simulink model "Vehicle_kinematics_model"  (R2017b)
settings: Solver=FixedStepAuto  StartTime=0.0  StopTime=10.0  FixedStep=0.01  RelTol=1e-3
settings Model: Creator=18428  LastModifiedBy=18428

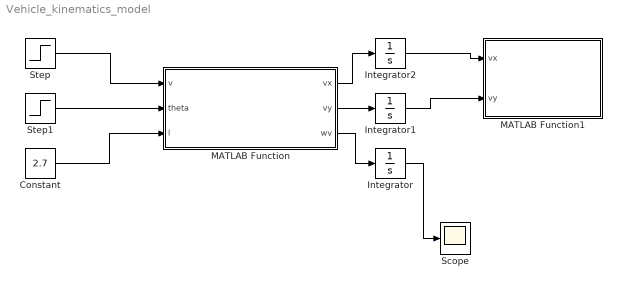
== system Vehicle_kinematics_model ==
  Constant : Constant  Value=2.7
  Integrator : Integrator
  Integrator1 : Integrator
  Integrator2 : Integrator
  MATLAB Function : MATLAB Function  TreatAsAtomicUnit=on
  MATLAB Function1 : MATLAB Function  TreatAsAtomicUnit=on
  Scope : Scope
  Step : Step  Time=0  After=5  SampleTime=0
  Step1 : Step  After=45  SampleTime=0
  wires:
  Step1/1 -> MATLAB Function/2(theta)
  Step/1 -> MATLAB Function/1(v)
  Constant/1 -> MATLAB Function/3(l)
  MATLAB Function/3(wv) -> Integrator/1
  Integrator/1 -> Scope/1
  MATLAB Function/2(vy) -> Integrator1/1
  MATLAB Function/1(vx) -> Integrator2/1
  Integrator2/1 -> MATLAB Function1/1(vx)
  Integrator1/1 -> MATLAB Function1/2(vy)

== matlab function Vehicle_kinematics_model/MATLAB Function1 ==
  data: vx input; vy input
function display_v(vx,vy)
    plot(vx,vy,'*');
    hold on
end

== matlab function Vehicle_kinematics_model/MATLAB Function ==
  data: v input; vx output; theta input; l input; vy output; wv output
function [vx,vy,wv] = Vehicle_kinematics_model(v,theta,l)
% v:速度
% theta:前轮偏角
% l:轴距
% vx:x方向速度
% vy:y方向速度
% wv:横摆角速度
degree2rad=pi/180;
w_rad = v*tan(theta*degree2rad/l);
vx = v*cos(w_rad);
vy = v*sin(w_rad);
wv = w_rad;
end
